simulink model "sim11b"  (R2015a)
settings: Solver=ode45  StartTime=0.0  StopTime=10.0  RelTol=1e-3
values from neighbouring files (symbols this model uses):
  k1 = 1/yl    (= 20)    [lab2.m]
  k2 = sqrt(2*k1)    [lab2.m]
settings Model: Creator=Pedro  LastModifiedBy=Pedro

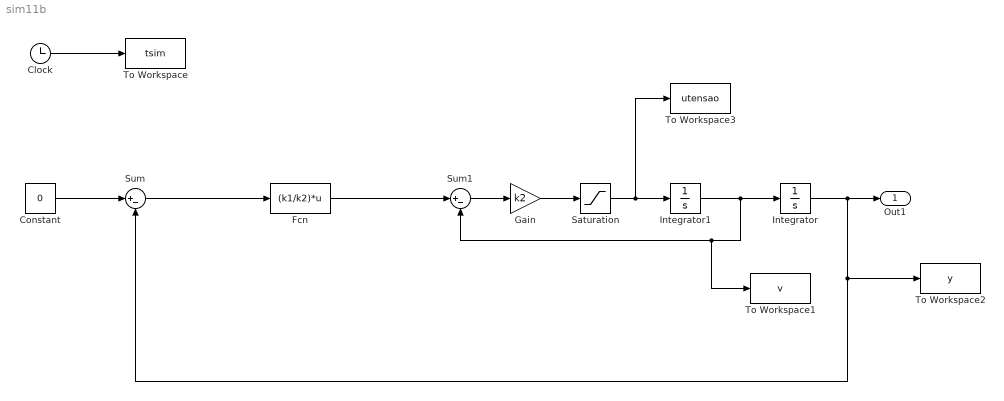
== system sim11b ==
  Clock : Clock
  Constant : Constant  Value=0
  Fcn : Fcn  Expr=(k1/k2)*u
  Gain : Gain  Gain=k2
  Integrator : Integrator  InitialCondition=1
  Integrator1 : Integrator
  Saturation : Saturate  UpperLimit=1  LowerLimit=-1
  Sum : Sum  Inputs=|+-
  Sum1 : Sum  Inputs=|+-
  To Workspace : ToWorkspace  VariableName=tsim  SampleTime=-1
  To Workspace1 : ToWorkspace  VariableName=v  SampleTime=-1
  To Workspace2 : ToWorkspace  VariableName=y  SampleTime=-1
  To Workspace3 : ToWorkspace  VariableName=utensao  SampleTime=-1
  Out1 : Outport
  wires:
  Sum1/1 -> Gain/1
  Gain/1 -> Saturation/1
  Saturation/1 -> To Workspace3/1, Integrator1/1
  Integrator1/1 -> To Workspace1/1, Sum1/2, Integrator/1
  Constant/1 -> Sum/1
  Integrator/1 -> To Workspace2/1, Sum/2, Out1/1
  Clock/1 -> To Workspace/1
  Fcn/1 -> Sum1/1
  Sum/1 -> Fcn/1
